simulink model "gps_simulate_24sat_demo"  (Simulink 7.3)
settings: Solver=ode45  StartTime=0.0  StopTime=86400  RelTol=1e-3
undefined symbols (not defined in the file): WGS
libraries: rapidstm32_gps_lib x5
settings Model: Creator=Compaq  LastModifiedBy=Compaq

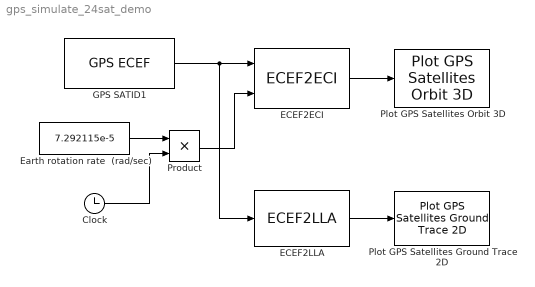
== system gps_simulate_24sat_demo ==
  Clock : Clock
      settings: Decimation=10
  ECEF2ECI : rapidstm32_gps_lib/ECEF2ECI
  ECEF2LLA : rapidstm32_gps_lib/ECEF2LLA  latlong_format=Degrees  altitude_format=Meters  refellipsoid=WGS-84  re=6378137  epsilon=0.081819190842622
  Earth rotation rate  (rad/sec) : Constant  Value=7.292115e-5  OutDataType=fixdt(1, 16)  OutScaling=2^0
  GPS SATID1 : rapidstm32_gps_lib/GPS ECEF  satid=All 24  t0=0  sampletime=600
  Plot GPS Satellites Ground Trace 2D : rapidstm32_gps_lib/Plot GPS Satellites Ground Trace 2D  satid_all=on  satid1=on  satid2=on  satid3=on  satid4=on  satid5=on  satid6=on  satid7=on  satid8=on  satid9=on  satid10=on  satid11=on  satid12=on  satid13=on  satid14=on  satid15=on  satid16=on  satid17=on  satid18=on  satid19=on  satid20=on  satid21=on  satid22=on  satid23=on  satid24=on  visibility_vec=No
  Plot GPS Satellites Orbit 3D : rapidstm32_gps_lib/Plot GPS Satellites Orbit 3D  satid_all=on  satid1=on  satid2=on  satid3=on  satid4=on  satid5=on  satid6=on  satid7=on  satid8=on  satid9=on  satid10=on  satid11=on  satid12=on  satid13=on  satid14=on  satid15=on  satid16=on  satid17=on  satid18=on  satid19=on  satid20=on  satid21=on  satid22=on  satid23=on  satid24=on  visibility_vec=No
  Product : Product  OutDataType=fixdt(1, 16)  OutScaling=2^0  RndMeth=Zero
  wires:
  Earth rotation rate  (rad/sec)/1 -> Product/1
  Clock/1 -> Product/2
  GPS SATID1/1 -> ECEF2ECI/1, ECEF2LLA/1
  Product/1 -> ECEF2ECI/2
  ECEF2ECI/1 -> Plot GPS Satellites Orbit 3D/1
  ECEF2LLA/1 -> Plot GPS Satellites Ground Trace 2D/1
